simulink model "ackerman_ROS_neural_controller_v2"  (R2023a)
settings: Solver=FixedStepDiscrete  StartTime=0.0  StopTime=200  FixedStep=0.1  RelTol=1e-3
undefined symbols (not defined in the file or in its folder): Angular, Linear
libraries: neural x413, robotlib x15, robotcorelib x1
(part 12 of 17)

== system ackerman_ROS_neural_controller_v2/casi 3 - 15 20 15/Layer 3/LW{3,2} ==
  "ad{3,2}" : Inport  PortDimensions=20  SampleTime=0.1
      mask Display: e = 0.06;c1 = [120 230 180]/255;c2 = ([120 230 180]+0)/(256+128);c3 = ([120 230 180]+128)/(256+128);patch([0 1 1 0],[0 0 1 1],c1);patch([0 1 1 1-e 1-e 0+e],[0 0 1 1-e 0+e 0+e],c2);patch([0 0 1 1-e 0+e 0+e],[0 1 1 1-e 1-e 0+e],c3);plot([0 1 1 0 0],[0 0 1 1 0]);
  "IW{3,2}(1,:)'" : Constant  Value=[-1.0099461495058019711024144271505065262317657470703125;0.89773679931498107098519767532707192003726959228515625;1.648022527449314100778110514511354267597198486328125;0.1868267631605853018594842751554097048938274383544921875;0.4326155427155338184519450805964879691600799560546875;-2.365931947396803902705642030923627316951751708984375;1.3131718941175243298147279347176663577556610107421875;-0.47831015230612639044238676433451473712921142578125;0.0187095015012974479062801691497952560894191265106201171875;0.253391071043920723671050154734984971582889556884765625;0.1711498827145969958696269941356149502098560333251953125;0.2105713055500454122803688505882746540009975433349609375;1.9992795560260088194581840070895850658416748046875;-0.551595982333906942329804223845712840557098388671875;0.904867215779645572837353029171936213970184326171875;0.2063587407911326720988398619738291017711162567138671875;-0.348442021104406085552085414747125469148159027099609375;1.0580412374047536427923432711395435035228729248046875;-1.7995275590595072312538604819565080106258392333984375;0.87988534548188279682534584935638122260570526123046875]
      mask Display: e = 0.06;c1 = [120 150 230]/255;c2 = ([120 150 230]+0)/383;c3 = ([120 150 230]+128)/383;patch([0 1 1 0],[0 0 1 1],c1);patch([0 1 1 1-e 1-e 0+e],[0 0 1 1-e 0+e 0+e],c2);patch([0 0 1 1-e 0+e 0+e],[0 1 1 1-e 1-e 0+e],c3);plot([0 1 1 0 0],[0 0 1 1 0]);disp('weights');
  "IW{3,2}(10,:)'" : Constant  Value=[0.449508971334619145121536121223471127450466156005859375;-1.69064901347178686563665905850939452648162841796875;-0.5625756471206810882534909978858195245265960693359375;-0.76668558865885361175429579816409386694431304931640625;1.137168314738134622388088246225379407405853271484375;0.1438794930428903828811826315359212458133697509765625;-1.7913778622428357945040033882833085954189300537109375;0.218615361461609036819453422140213660895824432373046875;0.84560267335105387953575473147793672978878021240234375;0.259066401169027515916098991510807536542415618896484375;-0.1681479147149977648734164858979056589305400848388671875;0.32783076605155525573565000740927644073963165283203125;-0.62425844223558912826632649739622138440608978271484375;-1.8918016159128416830981223029084503650665283203125;-0.257218110882138029094079456626786850392818450927734375;-0.47026275247000504098338069525198079645633697509765625;1.134036298735985770491652147029526531696319580078125;-1.782940942961468433480831663473509252071380615234375;0.448271013816211316704851697068079374730587005615234375;0.012596405616517140912957728460241924040019512176513671875]
      mask Display: e = 0.06;c1 = [120 150 230]/255;c2 = ([120 150 230]+0)/383;c3 = ([120 150 230]+128)/383;patch([0 1 1 0],[0 0 1 1],c1);patch([0 1 1 1-e 1-e 0+e],[0 0 1 1-e 0+e 0+e],c2);patch([0 0 1 1-e 0+e 0+e],[0 1 1 1-e 1-e 0+e],c3);plot([0 1 1 0 0],[0 0 1 1 0]);disp('weights');
  "IW{3,2}(11,:)'" : Constant  Value=[0.70657639702599095432589137999457307159900665283203125;0.26315953744514342105276227812282741069793701171875;-1.5325454973655390222830874336068518459796905517578125;0.2309244394443312753395503023057244718074798583984375;-0.4407827529243315556328752791159786283969879150390625;0.104508520200013610423894760970142669975757598876953125;0.373244624954732984178917831741273403167724609375;0.4116261193974370957704422835377044975757598876953125;0.71788504743435621602287710629752837121486663818359375;-1.7097691901798184321847884348244406282901763916015625;-0.303895752487840675737373885567649267613887786865234375;-2.36195872168838150173542089760303497314453125;0.38350240549765246544922092652996070683002471923828125;-0.273335251937565748558967015924281440675258636474609375;-1.2421889624792405992792510005529038608074188232421875;0.1718905030897595331840221888342057354748249053955078125;0.044644066652688031704432347623878740705549716949462890625;-0.802088031777856258486281149089336395263671875;-0.91419130941052006988911671214736998081207275390625;-1.3468214345745812554611120503977872431278228759765625]
      mask Display: e = 0.06;c1 = [120 150 230]/255;c2 = ([120 150 230]+0)/383;c3 = ([120 150 230]+128)/383;patch([0 1 1 0],[0 0 1 1],c1);patch([0 1 1 1-e 1-e 0+e],[0 0 1 1-e 0+e 0+e],c2);patch([0 0 1 1-e 0+e 0+e],[0 1 1 1-e 1-e 0+e],c3);plot([0 1 1 0 0],[0 0 1 1 0]);disp('weights');
  "IW{3,2}(12,:)'" : Constant  Value=[2.34324865740917598344594807713292539119720458984375;-0.2456791295145859255200093684834428131580352783203125;-0.62511000058684518254636941492208279669284820556640625;-0.160230805138303455947834663675166666507720947265625;-0.7414819526891260892398349824361503124237060546875;0.686580748353167624742354746558703482151031494140625;-2.482903758914255742951127103879116475582122802734375;1.706457578109262129828493925742805004119873046875;1.2638512279030986729111418753745965659618377685546875;-0.43081530832278336351492953326669521629810333251953125;-0.95519238768506287140525046197581104934215545654296875;0.864744929841261722458511940203607082366943359375;0.95051632746179126609575860129552893340587615966796875;1.33825141983004325396677813841961324214935302734375;0.88790396888644573802906734272255562245845794677734375;-1.259991486447709529983285392518155276775360107421875;-0.57048155058160665564770397395477630198001861572265625;-1.8187169461654788538140792297781445086002349853515625;1.316078828622404994774797160062007606029510498046875;-2.38968457127881617196862862328998744487762451171875]
      mask Display: e = 0.06;c1 = [120 150 230]/255;c2 = ([120 150 230]+0)/383;c3 = ([120 150 230]+128)/383;patch([0 1 1 0],[0 0 1 1],c1);patch([0 1 1 1-e 1-e 0+e],[0 0 1 1-e 0+e 0+e],c2);patch([0 0 1 1-e 0+e 0+e],[0 1 1 1-e 1-e 0+e],c3);plot([0 1 1 0 0],[0 0 1 1 0]);disp('weights');
  "IW{3,2}(13,:)'" : Constant  Value=[-0.1881084031898996034026794177407282404601573944091796875;-0.34153604634548118124115489990799687802791595458984375;-0.7506885441118438251351108192466199398040771484375;-0.80369662981443046323448697876301594078540802001953125;-1.2604035511614883890985083780833519995212554931640625;0.953889364010645834923707298003137111663818359375;0.51789220170325667158550686508533544838428497314453125;0.1603300753774819231711745715074357576668262481689453125;0.6851573303528606384560362130287103354930877685546875;0.8698064571084900276076723457663320004940032958984375;-0.64908030046581044469888865933171473443508148193359375;-0.07176839339938301254306907139834947884082794189453125;-0.61275798627052202594001073521212674677371978759765625;-1.010401401214933603256440619588829576969146728515625;0.213015572092948690663405386658268980681896209716796875;0.366504830544816417869924407568760216236114501953125;-0.3902350055952144014526083992677740752696990966796875;-0.891795645962334848633190631517209112644195556640625;-0.2109438517948613867059037829676526598632335662841796875;0.427886112564190679297126962410402484238147735595703125]
      mask Display: e = 0.06;c1 = [120 150 230]/255;c2 = ([120 150 230]+0)/383;c3 = ([120 150 230]+128)/383;patch([0 1 1 0],[0 0 1 1],c1);patch([0 1 1 1-e 1-e 0+e],[0 0 1 1-e 0+e 0+e],c2);patch([0 0 1 1-e 0+e 0+e],[0 1 1 1-e 1-e 0+e],c3);plot([0 1 1 0 0],[0 0 1 1 0]);disp('weights');
  "IW{3,2}(14,:)'" : Constant  Value=[-0.00935612807173313680564330496736147324554622173309326171875;-0.2327488199663734491640099122378160245716571807861328125;-1.015129383202438617672669352032244205474853515625;-0.4586085693356503067974472287460230290889739990234375;1.0921616645258367395143750400166027247905731201171875;-0.6736429053316015380659109723637811839580535888671875;1.0618488694554830686911373049952089786529541015625;0.34129227961505115285234523980761878192424774169921875;0.06335399477223868647257631891989149153232574462890625;-0.2699671046508200777935826408793218433856964111328125;0.6766261415525580691365803431835956871509552001953125;-1.8567942733653908238267149499733932316303253173828125;-0.376296268866221417237483137796516530215740203857421875;1.68994778775957765759585527121089398860931396484375;0.7492175070583011464719902505748905241489410400390625;0.33280430155064077979432113352231681346893310546875;0.299841077547019996263344410181161947548389434814453125;1.6860722591466912323454607758321799337863922119140625;0.290648698400503391336968661562423221766948699951171875;0.412387438008683882006977228229516185820102691650390625]
      mask Display: e = 0.06;c1 = [120 150 230]/255;c2 = ([120 150 230]+0)/383;c3 = ([120 150 230]+128)/383;patch([0 1 1 0],[0 0 1 1],c1);patch([0 1 1 1-e 1-e 0+e],[0 0 1 1-e 0+e 0+e],c2);patch([0 0 1 1-e 0+e 0+e],[0 1 1 1-e 1-e 0+e],c3);plot([0 1 1 0 0],[0 0 1 1 0]);disp('weights');
  "IW{3,2}(15,:)'" : Constant  Value=[-0.37193637695957149080783210592926479876041412353515625;0.0300266139736714531005556949594392790459096431732177734375;-1.539733439623463429057892426499165594577789306640625;0.1562279013691011131381713994414894841611385345458984375;-1.0028584795924835315616974185104481875896453857421875;0.8197804007340099285983114896225742995738983154296875;1.0464452267453470124536352159339003264904022216796875;0.31713285283596059915822706898325122892856597900390625;-1.989103976921534400190694213961251080036163330078125;1.84970673874586655216489816666580736637115478515625;-0.028510726678116930787876270869674044661223888397216796875;-0.06273844458487128072921024113384191878139972686767578125;2.304691563610864246669507338083349168300628662109375;0.2493512576221034449108771013925434090197086334228515625;-1.38784027881610949606283611501567065715789794921875;0.2234490960702558981498810908306040801107883453369140625;0.686438253270745146750186904682777822017669677734375;-1.099829554471054127162688018870539963245391845703125;-1.09744863031443795620134551427327096462249755859375;-0.190506591657872037526288977460353635251522064208984375]
      mask Display: e = 0.06;c1 = [120 150 230]/255;c2 = ([120 150 230]+0)/383;c3 = ([120 150 230]+128)/383;patch([0 1 1 0],[0 0 1 1],c1);patch([0 1 1 1-e 1-e 0+e],[0 0 1 1-e 0+e 0+e],c2);patch([0 0 1 1-e 0+e 0+e],[0 1 1 1-e 1-e 0+e],c3);plot([0 1 1 0 0],[0 0 1 1 0]);disp('weights');
  "IW{3,2}(2,:)'" : Constant  Value=[-0.326416616751357968606583881410188041627407073974609375;0.2151657967886707323312833750605932436883449554443359375;0.456374269952072975087276063277386128902435302734375;0.1569937653965003121481203152143280021846294403076171875;-0.48718134918667554966731358945253305137157440185546875;0.206551494625166476293287587395752780139446258544921875;-0.5857135921569456282753662890172563493251800537109375;-1.2183460272808031010782769953948445618152618408203125;0.43684346042053057157517059749807231128215789794921875;0.145108582453530476907843649314600042998790740966796875;2.581654038247091609292738212388940155506134033203125;0.1301568649229671581490919152201968245208263397216796875;-1.94621729841558543938617731328122317790985107421875;-0.4598080814387461856540539884008467197418212890625;-1.06112609605181074101665217312984168529510498046875;0.2011459035861979105508368093069293536245822906494140625;-1.134328654162411798012044528149999678134918212890625;2.050391425135473344454339894582517445087432861328125;1.5802886086008343102804474256117828190326690673828125;-0.0225650446991754079217873396601135027594864368438720703125]
      mask Display: e = 0.06;c1 = [120 150 230]/255;c2 = ([120 150 230]+0)/383;c3 = ([120 150 230]+128)/383;patch([0 1 1 0],[0 0 1 1],c1);patch([0 1 1 1-e 1-e 0+e],[0 0 1 1-e 0+e 0+e],c2);patch([0 0 1 1-e 0+e 0+e],[0 1 1 1-e 1-e 0+e],c3);plot([0 1 1 0 0],[0 0 1 1 0]);disp('weights');
  "IW{3,2}(3,:)'" : Constant  Value=[-1.1155611193286631976917533393134362995624542236328125;0.6011132957884972594087003017193637788295745849609375;0.638761123212283177252857058192603290081024169921875;0.8668650007290572556684082883293740451335906982421875;-0.354916334626522722572872226010076701641082763671875;-0.799552612390611816550745061249472200870513916015625;-0.77000621655026380008024489143281243741512298583984375;-0.986065464590628604213407015777193009853363037109375;-1.20799450083626513929857537732459604740142822265625;1.205789597555635861425571420113556087017059326171875;-0.15950145183662345349517863724031485617160797119140625;0.777115374860233298903722243267111480236053466796875;-0.0829669012759982338334197038420825265347957611083984375;-0.170132276933904369453642857479280792176723480224609375;0.22350431887964028465631827202741988003253936767578125;1.4492626155847248003993854581494815647602081298828125;-0.9820373755153199990530765717267058789730072021484375;-0.51424994532549284098621455996180884540081024169921875;-0.06760777759475104786712762461320380680263042449951171875;-1.1323905323416691981464055061223916709423065185546875]
      mask Display: e = 0.06;c1 = [120 150 230]/255;c2 = ([120 150 230]+0)/383;c3 = ([120 150 230]+128)/383;patch([0 1 1 0],[0 0 1 1],c1);patch([0 1 1 1-e 1-e 0+e],[0 0 1 1-e 0+e 0+e],c2);patch([0 0 1 1-e 0+e 0+e],[0 1 1 1-e 1-e 0+e],c3);plot([0 1 1 0 0],[0 0 1 1 0]);disp('weights');
  "IW{3,2}(4,:)'" : Constant  Value=[0.29763291600984598250789758822065778076648712158203125;-0.56529603972039677017846770468167960643768310546875;-0.8573623864163817387407107162289321422576904296875;-1.4983124672530951926319175981916487216949462890625;0.338392399317185621487880098356981761753559112548828125;2.49194325853409370807867162511684000492095947265625;1.52886728222341350402757598203606903553009033203125;-0.0662997178317719093598725521587766706943511962890625;-2.658175360622837768431736549246124923229217529296875;-0.046694118878899772140389501373647362925112247467041015625;0.88812217620468103529418613106827251613140106201171875;-0.81346700783210612595297561711049638688564300537109375;-0.77384462681643439996292954674572683870792388916015625;-0.0967264913508987522750004472982254810631275177001953125;0.144506771871039052523855161780375055968761444091796875;0.4062103455838457222171200555749237537384033203125;0.8095272899084211548625944487866945564746856689453125;-0.304869334813572534503833821872831322252750396728515625;-0.25933405342963211648310561940888874232769012451171875;-0.4690132770056483213494402662036009132862091064453125]
      mask Display: e = 0.06;c1 = [120 150 230]/255;c2 = ([120 150 230]+0)/383;c3 = ([120 150 230]+128)/383;patch([0 1 1 0],[0 0 1 1],c1);patch([0 1 1 1-e 1-e 0+e],[0 0 1 1-e 0+e 0+e],c2);patch([0 0 1 1-e 0+e 0+e],[0 1 1 1-e 1-e 0+e],c3);plot([0 1 1 0 0],[0 0 1 1 0]);disp('weights');
  "IW{3,2}(5,:)'" : Constant  Value=[0.2498753504496476207652477796727907843887805938720703125;-0.61876075038625166779837627473170869052410125732421875;-0.033983147267475720398888228146461187861859798431396484375;0.17323888778454199499634569292538799345493316650390625;-0.72442817063941300492757591200643219053745269775390625;0.5247832987458795894752938693272881209850311279296875;0.60573188465640626088060116671840660274028778076171875;-0.346533175761349288013235536709544248878955841064453125;-0.7178202933216386583126222831197082996368408203125;3.301749084004568235428678235621191561222076416015625;0.97923806650063494050328927187365479767322540283203125;0.70011998558531118863612618952174670994281768798828125;1.547616548977936989928139155381359159946441650390625;1.03505232833495153244030007044784724712371826171875;0.91947948277742297396031290190876461565494537353515625;-0.68036579123753482267744630007655359804630279541015625;0.65782070140286952319996771620935760438442230224609375;-0.147942219844305611342605288882623426616191864013671875;-1.29296079762602023066619949531741440296173095703125;-1.399249141413494879060408493387512862682342529296875]
      mask Display: e = 0.06;c1 = [120 150 230]/255;c2 = ([120 150 230]+0)/383;c3 = ([120 150 230]+128)/383;patch([0 1 1 0],[0 0 1 1],c1);patch([0 1 1 1-e 1-e 0+e],[0 0 1 1-e 0+e 0+e],c2);patch([0 0 1 1-e 0+e 0+e],[0 1 1 1-e 1-e 0+e],c3);plot([0 1 1 0 0],[0 0 1 1 0]);disp('weights');
  "IW{3,2}(6,:)'" : Constant  Value=[0.057681238475825791223172700483701191842555999755859375;-0.2487715055814197773198515051262802444398403167724609375;0.21639984209136942094886535414843820035457611083984375;0.1472882675437496846626572732930071651935577392578125;2.284170425385157354725151890306733548641204833984375;0.97421780446597150415755095309577882289886474609375;1.556357983477391737636708057834766805171966552734375;-0.436353531105683478674706066158250905573368072509765625;3.761063649019806387485687082516960799694061279296875;-1.0895138579235668085942734251148067414760589599609375;-0.93439642391536192889134326833300292491912841796875;-0.60298510363685864366090072508086450397968292236328125;-0.53527457577984682846050645821378566324710845947265625;-0.215355340249912485806049744496704079210758209228515625;2.78870887180425608420364369521848857402801513671875;0.8735886816703679613738131592981517314910888671875;0.296383929009733482207167298838612623512744903564453125;0.24650996087182075466870401214691810309886932373046875;-0.93328500489783972060564565254026092588901519775390625;1.67603276455609062622897909022867679595947265625]
      mask Display: e = 0.06;c1 = [120 150 230]/255;c2 = ([120 150 230]+0)/383;c3 = ([120 150 230]+128)/383;patch([0 1 1 0],[0 0 1 1],c1);patch([0 1 1 1-e 1-e 0+e],[0 0 1 1-e 0+e 0+e],c2);patch([0 0 1 1-e 0+e 0+e],[0 1 1 1-e 1-e 0+e],c3);plot([0 1 1 0 0],[0 0 1 1 0]);disp('weights');
  "IW{3,2}(7,:)'" : Constant  Value=[-0.62147323794078002112684089297545142471790313720703125;-0.2045909898130579829267361446909490041434764862060546875;1.0482839730530770783190064321388490498065948486328125;0.7816477428673109795198570282082073390483856201171875;-1.2265548256170897278849452050053514540195465087890625;1.4352949465045348187430818143184296786785125732421875;0.73769152560929907025411012000404298305511474609375;0.6018094295250080438819395567406900227069854736328125;-1.2966202644203008720324987734784372150897979736328125;-0.1850571436425703375494578040161286480724811553955078125;0.7937357021008464297295859068981371819972991943359375;-0.36933518189271641318782712914980947971343994140625;-0.455320722274156264308686559161287732422351837158203125;1.083913614942582537281623444869183003902435302734375;1.35952549183290738454843449289910495281219482421875;-1.8644400114256551859170940588228404521942138671875;-0.7841544767425332462806863986770622432231903076171875;0.334195733414011930673126471447176299989223480224609375;1.766306079640503678973573187249712646007537841796875;0.4919318874147344811120774465962313115596771240234375]
      mask Display: e = 0.06;c1 = [120 150 230]/255;c2 = ([120 150 230]+0)/383;c3 = ([120 150 230]+128)/383;patch([0 1 1 0],[0 0 1 1],c1);patch([0 1 1 1-e 1-e 0+e],[0 0 1 1-e 0+e 0+e],c2);patch([0 0 1 1-e 0+e 0+e],[0 1 1 1-e 1-e 0+e],c3);plot([0 1 1 0 0],[0 0 1 1 0]);disp('weights');
  "IW{3,2}(8,:)'" : Constant  Value=[-0.484332204095961504908274264380452223122119903564453125;0.06828409318236440539440224029021919704973697662353515625;-0.8190516986572002888777888074400834739208221435546875;0.406553837421733899049058891250751912593841552734375;-0.1088227821080836876799224910428165458142757415771484375;-0.460535304005593559839581985215772874653339385986328125;1.171188311470893861354625187232159078121185302734375;-0.63837668814209858059172120192670263350009918212890625;1.0762712142194035269682217403897084295749664306640625;1.2994660859712217071404438684112392365932464599609375;-0.484385526438760039003028623483260162174701690673828125;0.036319349078116403006788459606468677520751953125;-0.338465856628346994927625246418756432831287384033203125;-0.17465073079858617344228832735097967088222503662109375;-0.3485965845865319767682422025245614349842071533203125;-0.347855153030728836416329841085826046764850616455078125;0.282577495871144723782464325267937965691089630126953125;1.4706590072660257195735766799771226942539215087890625;0.54155059702517061026583178318105638027191162109375;-1.2864467445017258029338336200453341007232666015625]
      mask Display: e = 0.06;c1 = [120 150 230]/255;c2 = ([120 150 230]+0)/383;c3 = ([120 150 230]+128)/383;patch([0 1 1 0],[0 0 1 1],c1);patch([0 1 1 1-e 1-e 0+e],[0 0 1 1-e 0+e 0+e],c2);patch([0 0 1 1-e 0+e 0+e],[0 1 1 1-e 1-e 0+e],c3);plot([0 1 1 0 0],[0 0 1 1 0]);disp('weights');
  "IW{3,2}(9,:)'" : Constant  Value=[0.0788566863789341987445169479542528279125690460205078125;-0.92363939466933064892373295151628553867340087890625;0.908282135939205925723172185826115310192108154296875;-0.831700461757710396426546139991842210292816162109375;-0.4283610135378090877367185385082848370075225830078125;-0.042932574656631104781379093537907465361058712005615234375;-1.06987230896686735803768897312693297863006591796875;1.0637881786198022382450290024280548095703125;1.941071750902296333407548445393331348896026611328125;1.6249058458196257159755759857944212853908538818359375;0.121025005832648357984027143174898810684680938720703125;-0.66425009884913366331460338187753222882747650146484375;-1.33915212200457034441569703631103038787841796875;0.314585311436833159337567167312954552471637725830078125;1.08663132840931808686946169473230838775634765625;-1.20502514802789928438642164110206067562103271484375;0.53916907095101651581359192277886904776096343994140625;-0.2715268571677504905181876893038861453533172607421875;1.2811027274622792671010529375053010880947113037109375;0.450415503496343128109202780251507647335529327392578125]
      mask Display: e = 0.06;c1 = [120 150 230]/255;c2 = ([120 150 230]+0)/383;c3 = ([120 150 230]+128)/383;patch([0 1 1 0],[0 0 1 1],c1);patch([0 1 1 1-e 1-e 0+e],[0 0 1 1-e 0+e 0+e],c2);patch([0 0 1 1-e 0+e 0+e],[0 1 1 1-e 1-e 0+e],c3);plot([0 1 1 0 0],[0 0 1 1 0]);disp('weights');
  Mux : Mux  Inputs=15
      mask Display: e = 0.06;c1 = [120 150 230]/255;c2 = ([120 150 230]+0)/383;c3 = ([120 150 230]+128)/383;patch([0 1 1 0],[0 0 1 1],c1);patch([0 1 1 1-e 1-e 0+e],[0 0 1 1-e 0+e 0+e],c2);patch([0 0 1 1-e 0+e 0+e],[0 1 1 1-e 1-e 0+e],c3);plot([0 1 1 0 0],[0 0 1 1 0]);disp('Mux');
  dotprod{1..15} (15 alike) : neural/Weight Functions/dotprod
  "lz{3,2}" : Outport
      mask Display: e = 0.06;c1 = [120 230 180]/255;c2 = ([120 230 180]+0)/(256+128);c3 = ([120 230 180]+128)/(256+128);patch([0 1 1 0],[0 0 1 1],c1);patch([0 1 1 1-e 1-e 0+e],[0 0 1 1-e 0+e 0+e],c2);patch([0 0 1 1-e 0+e 0+e],[0 1 1 1-e 1-e 0+e],c3);plot([0 1 1 0 0],[0 0 1 1 0]);
  wires:
  "IW{3,2}(1,:)'"/1 -> dotprod1/1
  "ad{3,2}"/1 -> dotprod1/2, dotprod2/2, dotprod3/2, dotprod4/2, dotprod5/2, dotprod6/2, dotprod7/2, dotprod8/2, dotprod9/2, dotprod10/2, dotprod11/2, dotprod12/2, dotprod13/2, dotprod14/2, dotprod15/2
  dotprod1/1 -> Mux/1
  "IW{3,2}(2,:)'"/1 -> dotprod2/1
  dotprod2/1 -> Mux/2
  "IW{3,2}(3,:)'"/1 -> dotprod3/1
  dotprod3/1 -> Mux/3
  "IW{3,2}(4,:)'"/1 -> dotprod4/1
  dotprod4/1 -> Mux/4
  "IW{3,2}(5,:)'"/1 -> dotprod5/1
  dotprod5/1 -> Mux/5
  "IW{3,2}(6,:)'"/1 -> dotprod6/1
  dotprod6/1 -> Mux/6
  "IW{3,2}(7,:)'"/1 -> dotprod7/1
  dotprod7/1 -> Mux/7
  "IW{3,2}(8,:)'"/1 -> dotprod8/1
  dotprod8/1 -> Mux/8
  "IW{3,2}(9,:)'"/1 -> dotprod9/1
  dotprod9/1 -> Mux/9
  "IW{3,2}(10,:)'"/1 -> dotprod10/1
  dotprod10/1 -> Mux/10
  "IW{3,2}(11,:)'"/1 -> dotprod11/1
  dotprod11/1 -> Mux/11
  "IW{3,2}(12,:)'"/1 -> dotprod12/1
  dotprod12/1 -> Mux/12
  "IW{3,2}(13,:)'"/1 -> dotprod13/1
  dotprod13/1 -> Mux/13
  "IW{3,2}(14,:)'"/1 -> dotprod14/1
  dotprod14/1 -> Mux/14
  "IW{3,2}(15,:)'"/1 -> dotprod15/1
  dotprod15/1 -> Mux/15
  Mux/1 -> "lz{3,2}"/1

== system ackerman_ROS_neural_controller_v2/casi 3 - 15 20 15/Layer 4/Delays 1 ==
  "p{4}" : Inport  PortDimensions=15  SampleTime=0.1
      mask Display: e = 0.06;c1 = [120 230 180]/255;c2 = ([120 230 180]+0)/(256+128);c3 = ([120 230 180]+128)/(256+128);patch([0 1 1 0],[0 0 1 1],c1);patch([0 1 1 1-e 1-e 0+e],[0 0 1 1-e 0+e 0+e],c2);patch([0 0 1 1-e 0+e 0+e],[0 1 1 1-e 1-e 0+e],c3);plot([0 1 1 0 0],[0 0 1 1 0]);
  mux : Mux  Inputs=1
      mask Display: e = 0.06;c1 = [120 150 230]/255;c2 = ([120 150 230]+0)/383;c3 = ([120 150 230]+128)/383;patch([0 1 1 0],[0 0 1 1],c1);patch([0 1 1 1-e 1-e 0+e],[0 0 1 1-e 0+e 0+e],c2);patch([0 0 1 1-e 0+e 0+e],[0 1 1 1-e 1-e 0+e],c3);plot([0 1 1 0 0],[0 0 1 1 0]);disp('Mux')
  "pd{4,3}" : Outport
      mask Display: e = 0.06;c1 = [120 230 180]/255;c2 = ([120 230 180]+0)/(256+128);c3 = ([120 230 180]+128)/(256+128);patch([0 1 1 0],[0 0 1 1],c1);patch([0 1 1 1-e 1-e 0+e],[0 0 1 1-e 0+e 0+e],c2);patch([0 0 1 1-e 0+e 0+e],[0 1 1 1-e 1-e 0+e],c3);plot([0 1 1 0 0],[0 0 1 1 0]);
  wires:
  "p{4}"/1 -> mux/1
  mux/1 -> "pd{4,3}"/1

== system ackerman_ROS_neural_controller_v2/casi 3 - 15 20 15/Layer 4/LW{4,3} ==
  "ad{4,3}" : Inport  PortDimensions=15  SampleTime=0.1
      mask Display: e = 0.06;c1 = [120 230 180]/255;c2 = ([120 230 180]+0)/(256+128);c3 = ([120 230 180]+128)/(256+128);patch([0 1 1 0],[0 0 1 1],c1);patch([0 1 1 1-e 1-e 0+e],[0 0 1 1-e 0+e 0+e],c2);patch([0 0 1 1-e 0+e 0+e],[0 1 1 1-e 1-e 0+e],c3);plot([0 1 1 0 0],[0 0 1 1 0]);
  "IW{4,3}(1,:)'" : Constant  Value=[-0.413645202109023835124190782153164036571979522705078125;-0.035325415377830904350986429562908597290515899658203125;0.450924294603504638434543494440731592476367950439453125;-0.01516739731166885478408357101898218388669192790985107421875;0.04514597408204305828416380563794518820941448211669921875;-0.02884566390379135480959149617774528451263904571533203125;0.141226142774145635438998169775004498660564422607421875;0.82288063200564209864751319400966167449951171875;-0.09843320984459559552792740078075439669191837310791015625;0.175039401092785429359111049052444286644458770751953125;0.803987498387578103375972204958088696002960205078125;0.225548861931135824487881791355903260409832000732421875;-0.9075692450343677553092902599018998444080352783203125;0.11339992861258295364645931613267748616635799407958984375;0.2395278176693900473726017708031577058136463165283203125]
      mask Display: e = 0.06;c1 = [120 150 230]/255;c2 = ([120 150 230]+0)/383;c3 = ([120 150 230]+128)/383;patch([0 1 1 0],[0 0 1 1],c1);patch([0 1 1 1-e 1-e 0+e],[0 0 1 1-e 0+e 0+e],c2);patch([0 0 1 1-e 0+e 0+e],[0 1 1 1-e 1-e 0+e],c3);plot([0 1 1 0 0],[0 0 1 1 0]);disp('weights');
  "IW{4,3}(2,:)'" : Constant  Value=[-0.1077340626375372367728999734026729129254817962646484375;0.307988030074488439158386654526111669838428497314453125;-0.060110660273988758550700595151283778250217437744140625;-0.3310809978332465153272323732380755245685577392578125;0.269092877699381782807819263325654901564121246337890625;-0.0504045568867811100144393776645301841199398040771484375;0.143235391902499509253487985915853641927242279052734375;0.323304052588248402866355490914429537951946258544921875;0.38403956392235472083740432935883291065692901611328125;0.139170560758753503183271504894946701824665069580078125;0.285525581526583305258526479519787244498729705810546875;-0.07739948136161700631419080309569835662841796875;-0.373061456186915829658090615339460782706737518310546875;0.169384937710641725328031270692008547484874725341796875;0.21027146625423343007099674650817178189754486083984375]
      mask Display: e = 0.06;c1 = [120 150 230]/255;c2 = ([120 150 230]+0)/383;c3 = ([120 150 230]+128)/383;patch([0 1 1 0],[0 0 1 1],c1);patch([0 1 1 1-e 1-e 0+e],[0 0 1 1-e 0+e 0+e],c2);patch([0 0 1 1-e 0+e 0+e],[0 1 1 1-e 1-e 0+e],c3);plot([0 1 1 0 0],[0 0 1 1 0]);disp('weights');
  Mux : Mux  Inputs=2
      mask Display: e = 0.06;c1 = [120 150 230]/255;c2 = ([120 150 230]+0)/383;c3 = ([120 150 230]+128)/383;patch([0 1 1 0],[0 0 1 1],c1);patch([0 1 1 1-e 1-e 0+e],[0 0 1 1-e 0+e 0+e],c2);patch([0 0 1 1-e 0+e 0+e],[0 1 1 1-e 1-e 0+e],c3);plot([0 1 1 0 0],[0 0 1 1 0]);disp('Mux');
  dotprod1 : neural/Weight Functions/dotprod
  dotprod2 : neural/Weight Functions/dotprod
  "lz{4,3}" : Outport
      mask Display: e = 0.06;c1 = [120 230 180]/255;c2 = ([120 230 180]+0)/(256+128);c3 = ([120 230 180]+128)/(256+128);patch([0 1 1 0],[0 0 1 1],c1);patch([0 1 1 1-e 1-e 0+e],[0 0 1 1-e 0+e 0+e],c2);patch([0 0 1 1-e 0+e 0+e],[0 1 1 1-e 1-e 0+e],c3);plot([0 1 1 0 0],[0 0 1 1 0]);
  wires:
  "IW{4,3}(1,:)'"/1 -> dotprod1/1
  "ad{4,3}"/1 -> dotprod1/2, dotprod2/2
  dotprod1/1 -> Mux/1
  "IW{4,3}(2,:)'"/1 -> dotprod2/1
  dotprod2/1 -> Mux/2
  Mux/1 -> "lz{4,3}"/1

== system ackerman_ROS_neural_controller_v2/casi 4 - 16 21 16/Layer 1/Delays 1 ==
  "p{1}" : Inport  PortDimensions=8  SampleTime=0.1
      mask Display: e = 0.06;c1 = [120 230 180]/255;c2 = ([120 230 180]+0)/(256+128);c3 = ([120 230 180]+128)/(256+128);patch([0 1 1 0],[0 0 1 1],c1);patch([0 1 1 1-e 1-e 0+e],[0 0 1 1-e 0+e 0+e],c2);patch([0 0 1 1-e 0+e 0+e],[0 1 1 1-e 1-e 0+e],c3);plot([0 1 1 0 0],[0 0 1 1 0]);
  mux : Mux  Inputs=1
      mask Display: e = 0.06;c1 = [120 150 230]/255;c2 = ([120 150 230]+0)/383;c3 = ([120 150 230]+128)/383;patch([0 1 1 0],[0 0 1 1],c1);patch([0 1 1 1-e 1-e 0+e],[0 0 1 1-e 0+e 0+e],c2);patch([0 0 1 1-e 0+e 0+e],[0 1 1 1-e 1-e 0+e],c3);plot([0 1 1 0 0],[0 0 1 1 0]);disp('Mux')
  "pd{1,1}" : Outport
      mask Display: e = 0.06;c1 = [120 230 180]/255;c2 = ([120 230 180]+0)/(256+128);c3 = ([120 230 180]+128)/(256+128);patch([0 1 1 0],[0 0 1 1],c1);patch([0 1 1 1-e 1-e 0+e],[0 0 1 1-e 0+e 0+e],c2);patch([0 0 1 1-e 0+e 0+e],[0 1 1 1-e 1-e 0+e],c3);plot([0 1 1 0 0],[0 0 1 1 0]);
  wires:
  "p{1}"/1 -> mux/1
  mux/1 -> "pd{1,1}"/1

== system ackerman_ROS_neural_controller_v2/casi 4 - 16 21 16/Layer 1/IW{1,1} ==
  "pd{1,1}" : Inport  PortDimensions=8  SampleTime=0.1
      mask Display: e = 0.06;c1 = [120 230 180]/255;c2 = ([120 230 180]+0)/(256+128);c3 = ([120 230 180]+128)/(256+128);patch([0 1 1 0],[0 0 1 1],c1);patch([0 1 1 1-e 1-e 0+e],[0 0 1 1-e 0+e 0+e],c2);patch([0 0 1 1-e 0+e 0+e],[0 1 1 1-e 1-e 0+e],c3);plot([0 1 1 0 0],[0 0 1 1 0]);
  "IW{1,1}(1,:)'" : Constant  Value=[-0.352631993416327560453282785601913928985595703125;0.92449814439564581558528288951492868363857269287109375;1.1335810726600215048165409825742244720458984375;0.700587279346871927288020742707885801792144775390625;0.2730506300705386468763435914297588169574737548828125;-0.43135906105631616203055500591290183365345001220703125;-0.96353740004998600365837546632974408566951751708984375;0.021851704885061544458846327643186668865382671356201171875]
      mask Display: e = 0.06;c1 = [120 150 230]/255;c2 = ([120 150 230]+0)/383;c3 = ([120 150 230]+128)/383;patch([0 1 1 0],[0 0 1 1],c1);patch([0 1 1 1-e 1-e 0+e],[0 0 1 1-e 0+e 0+e],c2);patch([0 0 1 1-e 0+e 0+e],[0 1 1 1-e 1-e 0+e],c3);plot([0 1 1 0 0],[0 0 1 1 0]);disp('Weights');
  "IW{1,1}(10,:)'" : Constant  Value=[0.180118151587226382748241348963347263634204864501953125;1.112521489871254321002425058395601809024810791015625;0.58279963346284835434829574296600185334682464599609375;-0.41302256986097918289857489071437157690525054931640625;-0.7381464257148981911171858882880769670009613037109375;-1.286095677484809574053770120372064411640167236328125;0.49718734053732915878498488382319919764995574951171875;-0.73668421839423581243266880846931599080562591552734375]
      mask Display: e = 0.06;c1 = [120 150 230]/255;c2 = ([120 150 230]+0)/383;c3 = ([120 150 230]+128)/383;patch([0 1 1 0],[0 0 1 1],c1);patch([0 1 1 1-e 1-e 0+e],[0 0 1 1-e 0+e 0+e],c2);patch([0 0 1 1-e 0+e 0+e],[0 1 1 1-e 1-e 0+e],c3);plot([0 1 1 0 0],[0 0 1 1 0]);disp('Weights');
  "IW{1,1}(11,:)'" : Constant  Value=[-0.93018200947402729372726071233046241104602813720703125;-0.1187442356880928640006089835878810845315456390380859375;0.002096040714904818906549888168910911190323531627655029296875;1.45319649182477039772720672772265970706939697265625;0.139200758834054305612681901038740761578083038330078125;0.5565504964674177212913264156668446958065032958984375;0.8567875357344048037333550382754765450954437255859375;-0.79420156434819177970751979955821298062801361083984375]
      mask Display: e = 0.06;c1 = [120 150 230]/255;c2 = ([120 150 230]+0)/383;c3 = ([120 150 230]+128)/383;patch([0 1 1 0],[0 0 1 1],c1);patch([0 1 1 1-e 1-e 0+e],[0 0 1 1-e 0+e 0+e],c2);patch([0 0 1 1-e 0+e 0+e],[0 1 1 1-e 1-e 0+e],c3);plot([0 1 1 0 0],[0 0 1 1 0]);disp('Weights');
  "IW{1,1}(12,:)'" : Constant  Value=[-0.9694433365554300241484497746569104492664337158203125;0.67738443895128408467343206211808137595653533935546875;-0.66075002111317082675867595753516070544719696044921875;0.42158893852511136746130659957998432219028472900390625;0.2524045320248828883080705054453574120998382568359375;1.141256344687394896908472219365648925304412841796875;-0.5452014722526319356887825051671825349330902099609375;1.1026516862991007084104921887046657502651214599609375]
      mask Display: e = 0.06;c1 = [120 150 230]/255;c2 = ([120 150 230]+0)/383;c3 = ([120 150 230]+128)/383;patch([0 1 1 0],[0 0 1 1],c1);patch([0 1 1 1-e 1-e 0+e],[0 0 1 1-e 0+e 0+e],c2);patch([0 0 1 1-e 0+e 0+e],[0 1 1 1-e 1-e 0+e],c3);plot([0 1 1 0 0],[0 0 1 1 0]);disp('Weights');
  "IW{1,1}(13,:)'" : Constant  Value=[-1.1277869282321131283453041760367341339588165283203125;0.944089015784108642748151396517641842365264892578125;0.67613581210698103785006196631002239882946014404296875;0.226831473555220153315303832641802728176116943359375;0.393629745005038333971469910466112196445465087890625;0.8000587976488946484465714092948473989963531494140625;-0.24896458816908995093086787164793349802494049072265625;1.013173143266016040797694586217403411865234375]
      mask Display: e = 0.06;c1 = [120 150 230]/255;c2 = ([120 150 230]+0)/383;c3 = ([120 150 230]+128)/383;patch([0 1 1 0],[0 0 1 1],c1);patch([0 1 1 1-e 1-e 0+e],[0 0 1 1-e 0+e 0+e],c2);patch([0 0 1 1-e 0+e 0+e],[0 1 1 1-e 1-e 0+e],c3);plot([0 1 1 0 0],[0 0 1 1 0]);disp('Weights');
  "IW{1,1}(14,:)'" : Constant  Value=[-0.9659801042009268368104812907404266297817230224609375;0.1868133767076515516780688130893395282328128814697265625;0.41093615934043825621557743943412788212299346923828125;-0.057025737134231264946482298228147556073963642120361328125;0.8392697726072466668512106480193324387073516845703125;-0.442477985977679122431283076366526074707508087158203125;-0.94076272548704797937801913576549850404262542724609375;-0.94668868212912904436251437800819985568523406982421875]
      mask Display: e = 0.06;c1 = [120 150 230]/255;c2 = ([120 150 230]+0)/383;c3 = ([120 150 230]+128)/383;patch([0 1 1 0],[0 0 1 1],c1);patch([0 1 1 1-e 1-e 0+e],[0 0 1 1-e 0+e 0+e],c2);patch([0 0 1 1-e 0+e 0+e],[0 1 1 1-e 1-e 0+e],c3);plot([0 1 1 0 0],[0 0 1 1 0]);disp('Weights');
  "IW{1,1}(15,:)'" : Constant  Value=[-1.2284476593282633860582109264214523136615753173828125;0.3688445329657168425541158285341225564479827880859375;-0.73591304654182321254296539336792193353176116943359375;0.77746734166919850839150285537471063435077667236328125;-0.021951336611089854178313629518015659414231777191162109375;-0.592886199599444552177374134771525859832763671875;-0.048699683538942994953657716905581764876842498779296875;-1.101177710879512883224151664762757718563079833984375]
      mask Display: e = 0.06;c1 = [120 150 230]/255;c2 = ([120 150 230]+0)/383;c3 = ([120 150 230]+128)/383;patch([0 1 1 0],[0 0 1 1],c1);patch([0 1 1 1-e 1-e 0+e],[0 0 1 1-e 0+e 0+e],c2);patch([0 0 1 1-e 0+e 0+e],[0 1 1 1-e 1-e 0+e],c3);plot([0 1 1 0 0],[0 0 1 1 0]);disp('Weights');
  "IW{1,1}(16,:)'" : Constant  Value=[-0.7152482766377457057416222596657462418079376220703125;-0.313360255968531065118298784000216983258724212646484375;-0.35975791260693068540632566509884782135486602783203125;0.441004329826036711725834038588800467550754547119140625;-0.283748269724121537915806356977554969489574432373046875;1.2808540800888004174140633040224201977252960205078125;1.0416323705659367160336614688276313245296478271484375;0.43320303385815694952043486409820616245269775390625]
      mask Display: e = 0.06;c1 = [120 150 230]/255;c2 = ([120 150 230]+0)/383;c3 = ([120 150 230]+128)/383;patch([0 1 1 0],[0 0 1 1],c1);patch([0 1 1 1-e 1-e 0+e],[0 0 1 1-e 0+e 0+e],c2);patch([0 0 1 1-e 0+e 0+e],[0 1 1 1-e 1-e 0+e],c3);plot([0 1 1 0 0],[0 0 1 1 0]);disp('Weights');
  "IW{1,1}(2,:)'" : Constant  Value=[-1.338744318488829687652241773321293294429779052734375;-0.79627586096732205778181423738715238869190216064453125;-0.261657177046662192676507174837752245366573333740234375;0.719514007246797149264239124022424221038818359375;0.447194816927762028857529230663203634321689605712890625;-0.77173886784414669204323899975861422717571258544921875;0.81712020872704627105775898598949424922466278076171875;0.47803043852074778019556333674699999392032623291015625]
      mask Display: e = 0.06;c1 = [120 150 230]/255;c2 = ([120 150 230]+0)/383;c3 = ([120 150 230]+128)/383;patch([0 1 1 0],[0 0 1 1],c1);patch([0 1 1 1-e 1-e 0+e],[0 0 1 1-e 0+e 0+e],c2);patch([0 0 1 1-e 0+e 0+e],[0 1 1 1-e 1-e 0+e],c3);plot([0 1 1 0 0],[0 0 1 1 0]);disp('Weights');
  "IW{1,1}(3,:)'" : Constant  Value=[-1.1321638061855592294335792757919989526271820068359375;0.6815656673253285280367208542884327471256256103515625;1.118298319846591226678356179036200046539306640625;0.1723014867367313740498246943388949148356914520263671875;0.9589973121535473321586096062674187123775482177734375;1.0728717114333103932466428886982612311840057373046875;0.42933383295578797511637958450592122972011566162109375;0.348494006846479853489739753058529458940029144287109375]
      mask Display: e = 0.06;c1 = [120 150 230]/255;c2 = ([120 150 230]+0)/383;c3 = ([120 150 230]+128)/383;patch([0 1 1 0],[0 0 1 1],c1);patch([0 1 1 1-e 1-e 0+e],[0 0 1 1-e 0+e 0+e],c2);patch([0 0 1 1-e 0+e 0+e],[0 1 1 1-e 1-e 0+e],c3);plot([0 1 1 0 0],[0 0 1 1 0]);disp('Weights');
  "IW{1,1}(4,:)'" : Constant  Value=[-0.6294315956731513228561425421503372490406036376953125;-0.48365995992341803688674417571746744215488433837890625;0.1386788071189582749465074584804824553430080413818359375;0.89161557311172268125432083252235315740108489990234375;-0.9005539839607934471388261954416520893573760986328125;0.1744638150179445845733283704248606227338314056396484375;0.222477623468174900978056029998697340488433837890625;1.3546555218898423955664611639804206788539886474609375]
      mask Display: e = 0.06;c1 = [120 150 230]/255;c2 = ([120 150 230]+0)/383;c3 = ([120 150 230]+128)/383;patch([0 1 1 0],[0 0 1 1],c1);patch([0 1 1 1-e 1-e 0+e],[0 0 1 1-e 0+e 0+e],c2);patch([0 0 1 1-e 0+e 0+e],[0 1 1 1-e 1-e 0+e],c3);plot([0 1 1 0 0],[0 0 1 1 0]);disp('Weights');
  "IW{1,1}(5,:)'" : Constant  Value=[-0.35464615702145441122894453656044788658618927001953125;0.32704479688846699314552779469522647559642791748046875;-0.52914896415162149256872226033010520040988922119140625;-0.92490295661911370306285107290023006498813629150390625;-0.9986744225625259208101169861038215458393096923828125;-0.179322924603428912604385914164595305919647216796875;-0.25112511793216307776077655944391153752803802490234375;1.0056137747601312515399740732391364872455596923828125]
      mask Display: e = 0.06;c1 = [120 150 230]/255;c2 = ([120 150 230]+0)/383;c3 = ([120 150 230]+128)/383;patch([0 1 1 0],[0 0 1 1],c1);patch([0 1 1 1-e 1-e 0+e],[0 0 1 1-e 0+e 0+e],c2);patch([0 0 1 1-e 0+e 0+e],[0 1 1 1-e 1-e 0+e],c3);plot([0 1 1 0 0],[0 0 1 1 0]);disp('Weights');
  "IW{1,1}(6,:)'" : Constant  Value=[1.0916148833049721389443220687098801136016845703125;1.0745357444416441250467642021249048411846160888671875;-0.29761131773442617287628308986313641071319580078125;0.0766502214826846051121123082339181564748287200927734375;1.21379891859746624760418853838928043842315673828125;-0.86480512886551619278208136165631003677845001220703125;-0.522518034209447979065998879377730190753936767578125;0.1535897381381066961747450250186375342309474945068359375]
      mask Display: e = 0.06;c1 = [120 150 230]/255;c2 = ([120 150 230]+0)/383;c3 = ([120 150 230]+128)/383;patch([0 1 1 0],[0 0 1 1],c1);patch([0 1 1 1-e 1-e 0+e],[0 0 1 1-e 0+e 0+e],c2);patch([0 0 1 1-e 0+e 0+e],[0 1 1 1-e 1-e 0+e],c3);plot([0 1 1 0 0],[0 0 1 1 0]);disp('Weights');
  "IW{1,1}(7,:)'" : Constant  Value=[0.264321828948948844839605953893624246120452880859375;0.170127467546762944916594051392166875302791595458984375;-0.64008901574517473864744943057303316891193389892578125;1.047678637031950632518828570027835667133331298828125;1.3801555788731418861203792403102852404117584228515625;-0.72750422744682829989670835857396014034748077392578125;-0.275424703887971300542147901069256477057933807373046875;0.41277778057943426137654796548304148018360137939453125]
      mask Display: e = 0.06;c1 = [120 150 230]/255;c2 = ([120 150 230]+0)/383;c3 = ([120 150 230]+128)/383;patch([0 1 1 0],[0 0 1 1],c1);patch([0 1 1 1-e 1-e 0+e],[0 0 1 1-e 0+e 0+e],c2);patch([0 0 1 1-e 0+e 0+e],[0 1 1 1-e 1-e 0+e],c3);plot([0 1 1 0 0],[0 0 1 1 0]);disp('Weights');
  "IW{1,1}(8,:)'" : Constant  Value=[0.65871921154362300665496832152712158858776092529296875;0.74242772775773235860441445765900425612926483154296875;1.01235560803534507812173615093342959880828857421875;0.1015634556096570439986948031219071708619594573974609375;-0.71895056394998146931385463176411576569080352783203125;0.439659158984555931137805373509763740003108978271484375;1.1777492778622387081810529707581736147403717041015625;-0.34228710288230435043743682399508543312549591064453125]
      mask Display: e = 0.06;c1 = [120 150 230]/255;c2 = ([120 150 230]+0)/383;c3 = ([120 150 230]+128)/383;patch([0 1 1 0],[0 0 1 1],c1);patch([0 1 1 1-e 1-e 0+e],[0 0 1 1-e 0+e 0+e],c2);patch([0 0 1 1-e 0+e 0+e],[0 1 1 1-e 1-e 0+e],c3);plot([0 1 1 0 0],[0 0 1 1 0]);disp('Weights');
  "IW{1,1}(9,:)'" : Constant  Value=[-0.76834228050783426322567493116366676986217498779296875;0.88954163456792245678883546133874915540218353271484375;0.933500301173747271121783342096023261547088623046875;-0.275075965284508894281856328234425745904445648193359375;1.380909895551113653056063412805087864398956298828125;0.54677577040653846385254155393340624868869781494140625;0.0988073043112149829170220982632599771022796630859375;-0.211632233477003384169989885776885785162448883056640625]
      mask Display: e = 0.06;c1 = [120 150 230]/255;c2 = ([120 150 230]+0)/383;c3 = ([120 150 230]+128)/383;patch([0 1 1 0],[0 0 1 1],c1);patch([0 1 1 1-e 1-e 0+e],[0 0 1 1-e 0+e 0+e],c2);patch([0 0 1 1-e 0+e 0+e],[0 1 1 1-e 1-e 0+e],c3);plot([0 1 1 0 0],[0 0 1 1 0]);disp('Weights');
  Mux : Mux  Inputs=16
      mask Display: e = 0.06;c1 = [120 150 230]/255;c2 = ([120 150 230]+0)/383;c3 = ([120 150 230]+128)/383;patch([0 1 1 0],[0 0 1 1],c1);patch([0 1 1 1-e 1-e 0+e],[0 0 1 1-e 0+e 0+e],c2);patch([0 0 1 1-e 0+e 0+e],[0 1 1 1-e 1-e 0+e],c3);plot([0 1 1 0 0],[0 0 1 1 0]);disp('Mux');
  dotprod{1..16} (16 alike) : neural/Weight Functions/dotprod
  "iz{1,1}" : Outport
      mask Display: e = 0.06;c1 = [120 230 180]/255;c2 = ([120 230 180]+0)/(256+128);c3 = ([120 230 180]+128)/(256+128);patch([0 1 1 0],[0 0 1 1],c1);patch([0 1 1 1-e 1-e 0+e],[0 0 1 1-e 0+e 0+e],c2);patch([0 0 1 1-e 0+e 0+e],[0 1 1 1-e 1-e 0+e],c3);plot([0 1 1 0 0],[0 0 1 1 0]);
  wires:
  "IW{1,1}(1,:)'"/1 -> dotprod1/1
  "pd{1,1}"/1 -> dotprod1/2, dotprod2/2, dotprod3/2, dotprod4/2, dotprod5/2, dotprod6/2, dotprod7/2, dotprod8/2, dotprod9/2, dotprod10/2, dotprod11/2, dotprod12/2, dotprod13/2, dotprod14/2, dotprod15/2, dotprod16/2
  dotprod1/1 -> Mux/1
  "IW{1,1}(2,:)'"/1 -> dotprod2/1
  dotprod2/1 -> Mux/2
  "IW{1,1}(3,:)'"/1 -> dotprod3/1
  dotprod3/1 -> Mux/3
  "IW{1,1}(4,:)'"/1 -> dotprod4/1
  dotprod4/1 -> Mux/4
  "IW{1,1}(5,:)'"/1 -> dotprod5/1
  dotprod5/1 -> Mux/5
  "IW{1,1}(6,:)'"/1 -> dotprod6/1
  dotprod6/1 -> Mux/6
  "IW{1,1}(7,:)'"/1 -> dotprod7/1
  dotprod7/1 -> Mux/7
  "IW{1,1}(8,:)'"/1 -> dotprod8/1
  dotprod8/1 -> Mux/8
  "IW{1,1}(9,:)'"/1 -> dotprod9/1
  dotprod9/1 -> Mux/9
  "IW{1,1}(10,:)'"/1 -> dotprod10/1
  dotprod10/1 -> Mux/10
  "IW{1,1}(11,:)'"/1 -> dotprod11/1
  dotprod11/1 -> Mux/11
  "IW{1,1}(12,:)'"/1 -> dotprod12/1
  dotprod12/1 -> Mux/12
  "IW{1,1}(13,:)'"/1 -> dotprod13/1
  dotprod13/1 -> Mux/13
  "IW{1,1}(14,:)'"/1 -> dotprod14/1
  dotprod14/1 -> Mux/14
  "IW{1,1}(15,:)'"/1 -> dotprod15/1
  dotprod15/1 -> Mux/15
  "IW{1,1}(16,:)'"/1 -> dotprod16/1
  dotprod16/1 -> Mux/16
  Mux/1 -> "iz{1,1}"/1

== system ackerman_ROS_neural_controller_v2/casi 4 - 16 21 16/Layer 2/Delays 1 ==
  "p{2}" : Inport  PortDimensions=16  SampleTime=0.1
      mask Display: e = 0.06;c1 = [120 230 180]/255;c2 = ([120 230 180]+0)/(256+128);c3 = ([120 230 180]+128)/(256+128);patch([0 1 1 0],[0 0 1 1],c1);patch([0 1 1 1-e 1-e 0+e],[0 0 1 1-e 0+e 0+e],c2);patch([0 0 1 1-e 0+e 0+e],[0 1 1 1-e 1-e 0+e],c3);plot([0 1 1 0 0],[0 0 1 1 0]);
  mux : Mux  Inputs=1
      mask Display: e = 0.06;c1 = [120 150 230]/255;c2 = ([120 150 230]+0)/383;c3 = ([120 150 230]+128)/383;patch([0 1 1 0],[0 0 1 1],c1);patch([0 1 1 1-e 1-e 0+e],[0 0 1 1-e 0+e 0+e],c2);patch([0 0 1 1-e 0+e 0+e],[0 1 1 1-e 1-e 0+e],c3);plot([0 1 1 0 0],[0 0 1 1 0]);disp('Mux')
  "pd{2,1}" : Outport
      mask Display: e = 0.06;c1 = [120 230 180]/255;c2 = ([120 230 180]+0)/(256+128);c3 = ([120 230 180]+128)/(256+128);patch([0 1 1 0],[0 0 1 1],c1);patch([0 1 1 1-e 1-e 0+e],[0 0 1 1-e 0+e 0+e],c2);patch([0 0 1 1-e 0+e 0+e],[0 1 1 1-e 1-e 0+e],c3);plot([0 1 1 0 0],[0 0 1 1 0]);
  wires:
  "p{2}"/1 -> mux/1
  mux/1 -> "pd{2,1}"/1
